simulink model "Forcing_Moment"  (R2023a)
settings: Solver=VariableStepAuto  StartTime=0.0  StopTime=10.0  RelTol=1e-3
values from neighbouring files (symbols this model uses):
  Cl_alpha = 0.0959    [Roll_variables.mat]
  rho = 1.225    [Roll_variables.mat]
settings Model: Creator=kwood  LastModifiedBy=kwood

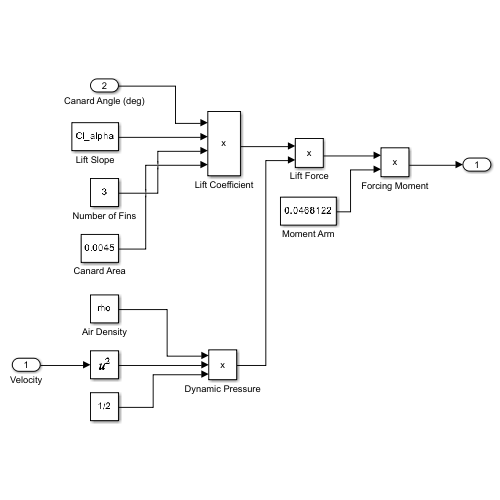
[thumbnail: Simulink's stored preview of the top-level diagram]
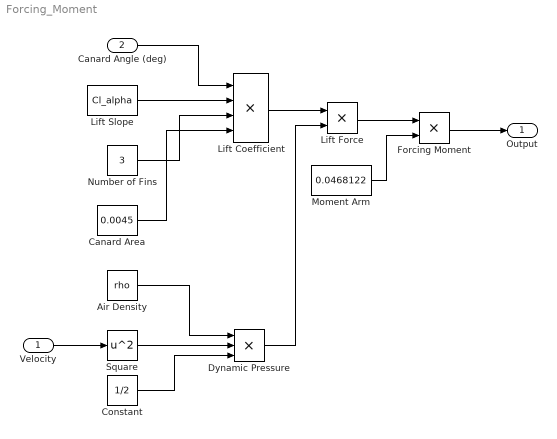
== system Forcing_Moment ==
  Velocity : Inport
  Canard Angle (deg) : Inport  Port=2
  Air Density : Constant  Value=rho
  Canard Area : Constant  Value=0.0045
  Constant : Constant  Value=1/2
  Dynamic Pressure : Product  Inputs=3
  Forcing Moment : Product
  Lift Coefficient : Product  Inputs=4
  Lift Force : Product
  Lift Slope : Constant  Value=Cl_alpha
  Moment Arm : Constant  Value=0.0468122
  Number of Fins : Constant  Value=3
  Square : Math  Operator=square
  Output : Outport
  wires:
  Lift Coefficient/1 -> Lift Force/1
  Velocity/1 -> Square/1
  Lift Slope/1 -> Lift Coefficient/2
  Canard Angle (deg)/1 -> Lift Coefficient/1
  Square/1 -> Dynamic Pressure/2
  Dynamic Pressure/1 -> Lift Force/2
  Air Density/1 -> Dynamic Pressure/1
  Canard Area/1 -> Lift Coefficient/4
  Number of Fins/1 -> Lift Coefficient/3
  Constant/1 -> Dynamic Pressure/3
  Forcing Moment/1 -> Output/1
  Lift Force/1 -> Forcing Moment/1
  Moment Arm/1 -> Forcing Moment/2
